simulink model "springsimu"  (R2019b)
settings: Solver=VariableStepAuto  StartTime=0.0  StopTime=10.0  RelTol=1e-3
settings Model: Creator=Admin  LastModifiedBy=Admin

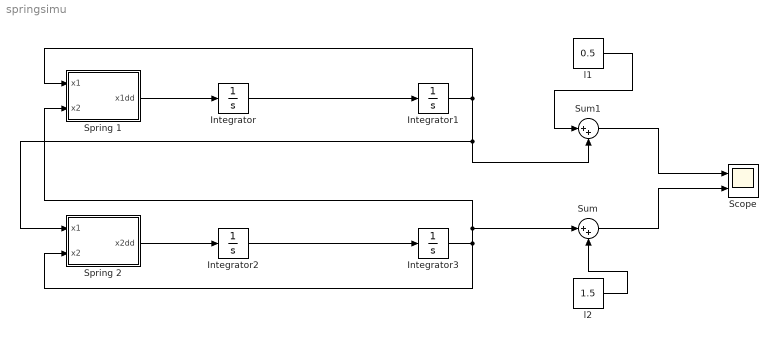
== system springsimu ==
  Integrator : Integrator
  Integrator1 : Integrator  InitialCondition=0.3
  Integrator2 : Integrator
  Integrator3 : Integrator  InitialCondition=0.7
  Scope : Scope  NumInputPorts=2
  Spring 1 : MATLAB Function  TreatAsAtomicUnit=on
  Spring 2 : MATLAB Function  TreatAsAtomicUnit=on
  Sum : Sum  Inputs=|++
  Sum1 : Sum  Inputs=|++
  l1 : Constant  Value=0.5
  l2 : Constant  Value=1.5
  wires:
  Integrator/1 -> Integrator1/1
  Spring 1/1(x1dd) -> Integrator/1
  Integrator1/1 -> Sum1/2, Spring 2/1(x1), Spring 1/1(x1)
  Integrator2/1 -> Integrator3/1
  Spring 2/1(x2dd) -> Integrator2/1
  Integrator3/1 -> Sum/1, Spring 1/2(x2), Spring 2/2(x2)
  l1/1 -> Sum1/1
  l2/1 -> Sum/2
  Sum1/1 -> Scope/1
  Sum/1 -> Scope/2

== matlab function springsimu/Spring 2 ==
  data: x1 input; x2dd output; x2 input
function x2dd = spring2(x1,x2)
m2=1;
%k1=2;
k2=4;
x2dd = (-k2*(x2-x1))/m2;

== matlab function springsimu/Spring 1 ==
  data: x1 input; x1dd output; x2 input
function x1dd = spring1(x1,x2)
m1=1;
k1=2;
k2=4;

x1dd = (k2*(x2-x1)-k1*x1)/m1;
